simulink model "noise"  (R2023a)
settings: Solver=VariableStepAuto  StartTime=0.0  StopTime=10.0  RelTol=1e-3
libraries: simulink x1
settings Model: Creator=xenja  LastModifiedBy=xenja

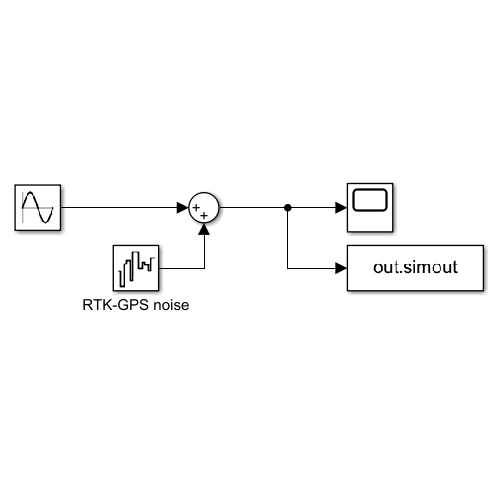
[thumbnail: Simulink's stored preview of the top-level diagram]
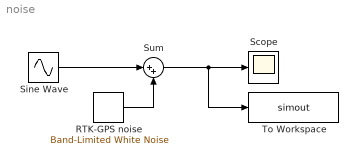
== system noise ==
  RTK-GPS noise : simulink/Sources/Band-Limited White Noise  Cov=[2.28]  Ts=0.1  seed=[23341]
  Scope : Scope
  Sine Wave : Sin  Amplitude=50  Frequency=(2*pi)*0.2  SampleTime=0
  Sum : Sum  Inputs=|++
  To Workspace : ToWorkspace  VariableName=simout  SaveFormat=Timeseries  SampleTime=-1
  wires:
  Sum/1 -> To Workspace/1, Scope/1
  Sine Wave/1 -> Sum/1
  RTK-GPS noise/1 -> Sum/2
